simulink model "sim2_80"  (R2023a)
settings: Solver=FixedStepAuto  StartTime=0.0  StopTime=0.001  FixedStep=dt  RelTol=dt
undefined symbols (not defined in the file): C, f2, L, R
settings Model: Creator=khald  LastModifiedBy=khald

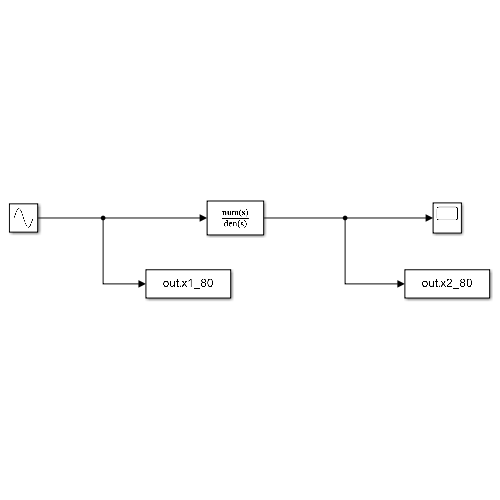
[thumbnail: Simulink's stored preview of the top-level diagram]
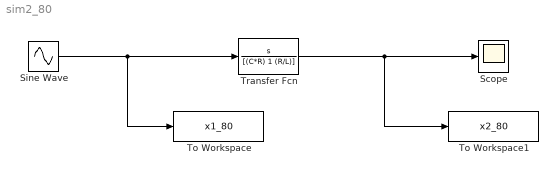
== system sim2_80 ==
  Scope : Scope
  Sine Wave : Sin  Frequency=f2  SampleTime=0
  To Workspace : ToWorkspace  VariableName=x1_80  SampleTime=-1
  To Workspace1 : ToWorkspace  VariableName=x2_80  SampleTime=-1
  Transfer Fcn : TransferFcn  Numerator=[1 0]  Denominator=[(C*R) 1 (R/L)]
  wires:
  Sine Wave/1 -> To Workspace/1, Transfer Fcn/1
  Transfer Fcn/1 -> To Workspace1/1, Scope/1
